simulink model "RL_fwd"  (R2014a)
settings: Solver=ode45  StartTime=0.0  StopTime=0.1  RelTol=1e-3
values from neighbouring files (symbols this model uses):
  alpha3 = e    [rl_fwd.m]
  f3 = b    [rl_fwd.m]
  l3 = d    [rl_fwd.m]
  r3 = c    [rl_fwd.m]
  v3 = a    [rl_fwd.m]
libraries: powerlib x10
settings Model: Creator=SAMBIT  LastModifiedBy=SAMBIT

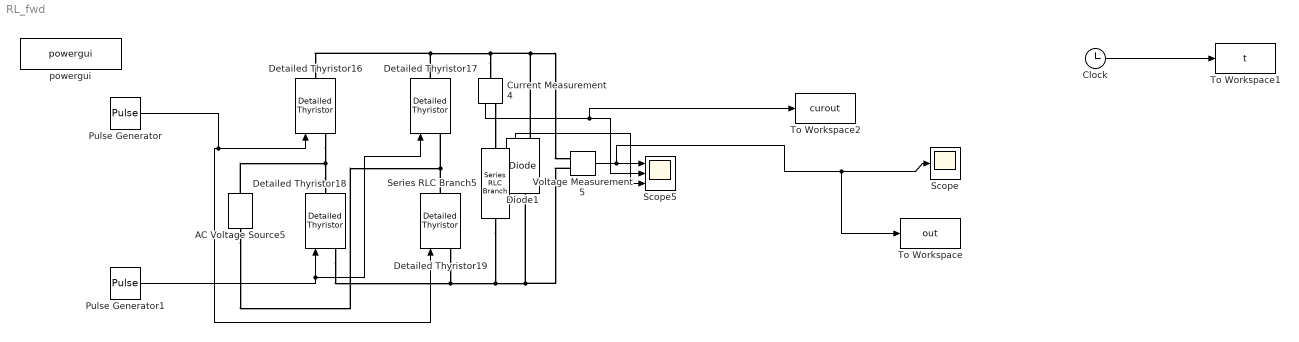
== system RL_fwd ==
  AC Voltage Source5 : powerlib/Electrical Sources/AC Voltage Source  Amplitude=v3  Phase=0  Frequency=f3  SampleTime=0  Measurements=None
  Clock : Clock
  Current Measurement4 : powerlib/Measurements/Current Measurement  PhasorSimulation=off  OutputType=Complex  PSBequivalent=0
  Detailed Thyristor16 : powerlib/Power Electronics/Detailed Thyristor  Ron=0.001  Lon=0  Vf=0.8  IL=0.1  Tq=1e-6  IC=0  Rs=500  Cs=1e-9  Measurements=off
  Detailed Thyristor17 : powerlib/Power Electronics/Detailed Thyristor  Ron=0.001  Lon=0  Vf=0  IL=0.1  Tq=1e-6  IC=0  Rs=500  Cs=1e-9  Measurements=off
  Detailed Thyristor18 : powerlib/Power Electronics/Detailed Thyristor  Ron=0.001  Lon=0  Vf=0  IL=0.1  Tq=1e-6  IC=0  Rs=500  Cs=1e-9  Measurements=off
  Detailed Thyristor19 : powerlib/Power Electronics/Detailed Thyristor  Ron=0.001  Lon=0  Vf=0.8  IL=0.1  Tq=1e-6  IC=0  Rs=500  Cs=1e-9  Measurements=off
  Diode1 : powerlib/Power Electronics/Diode  Ron=0.001  Lon=0  Vf=0.8  IC=0  UseSnubber=off  Rs=500  Cs=250e-9  Measurements=on
  Pulse Generator : DiscretePulseGenerator  PulseType=Time based  Period=1/f3  PulseWidth=5  PhaseDelay=((1/f3)/360)*alpha3
  Pulse Generator1 : DiscretePulseGenerator  PulseType=Time based  Period=1/f3  PulseWidth=5  PhaseDelay=(((1/f3)/360)*alpha3)+((1/f3)/2)
  Scope : Scope
  Scope5 : Scope  NumInputPorts=3
      settings: YMin=-5~-2~-5  YMax=105~14~5  SaveName=SPBR_HL_FD  MaxDataPoints=5000000  SampleInput=on  SampleTime=5e-6
  Series RLC Branch5 : powerlib/Elements/Series RLC Branch  LConnTagsString=__new0  RConnTagsString=__new0  BranchType=RL  Resistance=r3  Inductance=l3  SetiL0=off  InitialCurrent=0  Capacitance=1e-6  Setx0=off  InitialVoltage=0  Measurements=None
  To Workspace : ToWorkspace  VariableName=out  SampleTime=-1
  To Workspace1 : ToWorkspace  VariableName=t  SampleTime=-1
  To Workspace2 : ToWorkspace  VariableName=curout  SampleTime=-1
  Voltage Measurement5 : powerlib/Measurements/Voltage Measurement  PhasorSimulation=off  OutputType=Complex  PSBequivalent=0
  powergui : powerlib/powergui  Priority=1  SimulationMode=Continuous  SolverType=Tustin  SampleTime=5e-6  frequency=60  SPID=off  DisableSnubberDevices=off  DisableRonSwitches=off  DisableVfSwitches=off  SwTol=0  Interpol=off  DisplayEquations=off  Ts=0  methode=off  frequencyindice=60  Pbase=100e6  ErrMax=1e-4  Iterations=50  UnitsV=kV  UnitsW=MW  FunctionMessages=off  echomessages=off  HookPort=off  EnableUseOfTLC=off  x0status=blocks  RestoreLinks=warning  ResistiveCurrentMeasurement=off  Frange=[0:2:500]  Ylog=off  Xlog=on  ShowGrid=off  save=off  variable=ZData  structure=SPBR_R  ZoomFFT=off  StartTime=0.0  cycles=1  DisplayStyle=1  fundamental=100  FreqAxis=off  MaxFrequency=1000  frequencyindicesteady=1  RmsSteady=1  display=off
  wires:
  Pulse Generator/1 -> Detailed Thyristor16/1, Detailed Thyristor19/1
  Pulse Generator1/1 -> Detailed Thyristor17/1, Detailed Thyristor18/1
  Diode1/1 -> Scope5/3
  Current Measurement4/1 -> To Workspace2/1, Scope5/2
  Clock/1 -> To Workspace1/1
  Voltage Measurement5/1 -> To Workspace/1, Scope/1, Scope5/1
  connections:
  Detailed Thyristor17/LConn1 -- AC Voltage Source5/LConn1 -- Detailed Thyristor19/RConn1
  Voltage Measurement5/LConn2 -- Detailed Thyristor19/LConn1 -- Detailed Thyristor18/LConn1 -- Series RLC Branch5/RConn1 -- Diode1/LConn1
  Detailed Thyristor18/RConn1 -- AC Voltage Source5/RConn1 -- Detailed Thyristor16/LConn1
  Current Measurement4/LConn1 -- Detailed Thyristor17/RConn1 -- Detailed Thyristor16/RConn1 -- Diode1/RConn1 -- Voltage Measurement5/LConn1
  Current Measurement4/RConn1 -- Series RLC Branch5/LConn1
